simulink model "SimpleCPUCoolingSystem"  (R2024a)
settings: Solver=VariableStepAuto  StartTime=0.0  StopTime=12000  RelTol=1e-3  AbsTol=1e-3  EnableMultiTasking=on
PreLoadFcn:
  | % CPU fan
  | omega_vec = [2000, 2500, 3000]; % Shaft speed vector (rpm)
  | dp_vec = unique([linspace(0, 34.8, 20), 16.1, 24.5]); % Static pressure gain vector (Pa)
  | flow_rate_2000rpm = [
  |    29.0291
  |    26.8708
  |    22.4003
  |    16.0321
  |    11.8087
  |    10.7402
  |    10.3039
  |     9.2101
  |     5.2882
  |     0.001
  |     0.001
  |     0.001
  |     0.001
  |     0.001
  |     0.001
  |     0.001
  |     0.001
  |     0.001
  |     0.001
  |     0.001
  |     0.001
  |     0.001]; % Volumetric flow rate at 2000 rpm (l/min)
  | 
  | flow_rate_2500rpm = [
  |    44.1599
  |    43.4754
  |    41.8968
  |    37.6981
  |    31.3796
  |    25.5726
  |    22.0781
  |    20.5303
  |    19.7231
  |    19.1403
  |    18.9864
  |    17.7518
  |    15.0095
  |     9.9392
  |     3.0478
  |     0.001
  |     0.001
  |     0.001
  |     0.001
  |     0.001
  |     0.001
  |     0.001]; % Volumetric flow rate at 2500 rpm (l/min)
  | 
  | flow_rate_3000rpm = [
  |    62.7057
  |    61.7375
  |    60.1794
  |    58.1656
  |    54.8140
  |    49.9250
  |    43.8984
  |    39.0101
  | ... (+42 lines)
libraries: fl_lib x20, nesl_utility x4, SimscapeFluids_lib x1
(part 2 of 2)

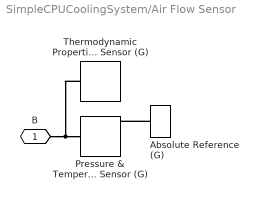
== system SimpleCPUCoolingSystem/Air Flow Sensor ==
  Absolute Reference (G) : fl_lib/Gas/Elements/Absolute Reference (G)
      settings: InternalSimscapePortConfiguration="{\"Bottom\":[],\"Left\":[{\"id\":\"A\",\"label\":\"\",\"type\":\"foundation.gas.gas\"}],\"Right\":[],\"Top\":[]}"
  Pressure & Temperature Sensor (G) : fl_lib/Gas/Sensors/Pressure & Temperature Sensor (G)  reference=foundation.enum.MeasurementReference.difference  pressure=true  pressure_spec=foundation.enum.PressureMeasementSpec.Absolute  temperature=true
      settings: InternalSimscapePortConfiguration="{\"Bottom\":[{\"id\":\"T\",\"label\":\"T\",\"type\":\"output\"}],\"Left\":[{\"id\":\"A\",\"label\":\"A\",\"type\":\"foundation.gas.gas\"}],\"Right\":[{\"id\":\"B\",\"label\":\"B\",\"type\":\"foundation.gas.gas\"},{\"id\":\"P\",\"label\":\"P\",\"type\":\"output\"}],\"Top\":[]}"
  Thermodynamic Properties Sensor (G) : fl_lib/Gas/Sensors/Thermodynamic Properties Sensor (G)  enthalpy=true  density=true  specific_heat=true  entropy=true  s_std=3.8635 kJ/kg/K  p_std=0.101325 MPa  T_std=293.15 K
      settings: InternalSimscapePortConfiguration="{\"Bottom\":[{\"id\":\"CP\",\"label\":\"cp\",\"type\":\"output\"},{\"id\":\"S\",\"label\":\"s\",\"type\":\"output\"}],\"Left\":[{\"id\":\"A\",\"label\":\"A\",\"type\":\"foundation.gas.gas\"}],\"Right\":[{\"id\":\"H\",\"label\":\"h\",\"type\":\"output\"},{\"id\":\"RHO\",\"label\":\"ρ\",\"type\":\"output\"}],\"Top\":[]}"
  B : PMIOPort  Side=Right
  connections:
  Absolute Reference (G)/LConn1 -- Pressure & Temperature Sensor (G)/RConn1
  B/RConn1 -- Thermodynamic Properties Sensor (G)/LConn1 -- Pressure & Temperature Sensor (G)/LConn1

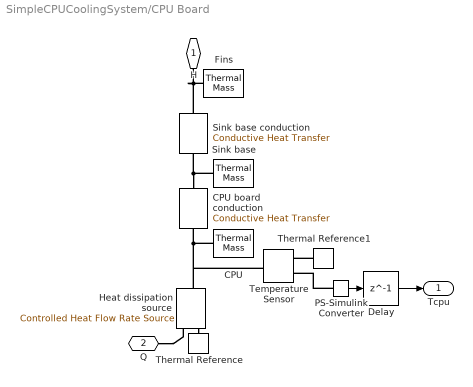
== system SimpleCPUCoolingSystem/CPU Board ==
  CPU : fl_lib/Thermal/Thermal Elements/Thermal Mass  mass_type=foundation.enum.constant_variable.constant  mass=rho_CPU*w_CPU^2*t_CPU g  sp_heat=cp_CPU J/kg/K  mass_min=1e-6 kg  num_ports=foundation.enum.numPorts2.one  m_specify=off  m_priority=High  m=1 kg  m_nominal_specify=off  m_nominal_value=1  m_nominal_unit=kg  T_specify=on  T_priority=High  T=T_init degC  T_nominal_specify=off  T_nominal_value=1  T_nominal_unit=K  Q_specify=off  Q_priority=None  Q=0 W  Q_nominal_specify=off  Q_nominal_value=1  Q_nominal_unit=W
  CPU board conduction : fl_lib/Thermal/Thermal Elements/Conductive Heat Transfer  thermal_type=foundation.enum.ConstantVariableTabulated.Constant  wall_geometry=foundation.enum.ConductionWallGeometry.Planar  area=w_CPU^2 cm^2  thickness=t_CPU cm  d_in=0.05 m  d_out=0.1 m  L=1 m  th_cond_min=10 W/(K*m)  th_cond=k_CPU W/(m*K)  th_cond_TLU=[413, 401, 392, 383, 371, 357, 342] W/(K*m)  temp_TLU=[200, 273, 400, 600, 800, 1000, 1200] K  T_specify=off  T_priority=None  T=0 K  T_nominal_specify=off  T_nominal_value=1  T_nominal_unit=K  Q_specify=off  Q_priority=None  Q=0 W  Q_nominal_specify=off  Q_nominal_value=1  Q_nominal_unit=W
  Delay : Delay  DelayLength=1  InitialCondition=T_init  SampleTime=30
  Fins : fl_lib/Thermal/Thermal Elements/Thermal Mass  mass_type=foundation.enum.constant_variable.constant  mass=rho_HS*N_Fin*t_Fin*h_Fin*l_Fin g  sp_heat=cp_HS J/kg/K  mass_min=1e-6 kg  num_ports=foundation.enum.numPorts2.one  m_specify=off  m_priority=High  m=1 kg  m_nominal_specify=off  m_nominal_value=1  m_nominal_unit=kg  T_specify=on  T_priority=High  T=T_init degC  T_nominal_specify=off  T_nominal_value=1  T_nominal_unit=K  Q_specify=off  Q_priority=None  Q=0 W  Q_nominal_specify=off  Q_nominal_value=1  Q_nominal_unit=W
  Heat dissipation source : fl_lib/Thermal/Thermal Sources/Controlled Heat Flow Rate Source
  PS-Simulink Converter : nesl_utility/PS-Simulink Converter  PhysicalDomain=network_engine_domain  SubClassName=ps_output  LeftPortType=input  RightPortType=output  PseudoPeriodic=off  Frequencies=[]  VectorFormat=1-D array  Unit=degC  AffineConversion=on
  Sink base : fl_lib/Thermal/Thermal Elements/Thermal Mass  mass_type=foundation.enum.constant_variable.constant  mass=rho_HS*w_HS^2*t_HS g  sp_heat=cp_HS J/kg/K  mass_min=1e-6 kg  num_ports=foundation.enum.numPorts2.one  m_specify=off  m_priority=High  m=1 kg  m_nominal_specify=off  m_nominal_value=1  m_nominal_unit=kg  T_specify=on  T_priority=High  T=T_init degC  T_nominal_specify=off  T_nominal_value=1  T_nominal_unit=K  Q_specify=off  Q_priority=None  Q=0 W  Q_nominal_specify=off  Q_nominal_value=1  Q_nominal_unit=W
  Sink base conduction : fl_lib/Thermal/Thermal Elements/Conductive Heat Transfer  thermal_type=foundation.enum.ConstantVariableTabulated.Constant  wall_geometry=foundation.enum.ConductionWallGeometry.Planar  area=N_Fin*l_Fin*t_Fin cm^2  thickness=t_HS cm  d_in=0.05 m  d_out=0.1 m  L=1 m  th_cond_min=10 W/(K*m)  th_cond=k_HS W/(m*K)  th_cond_TLU=[413, 401, 392, 383, 371, 357, 342] W/(K*m)  temp_TLU=[200, 273, 400, 600, 800, 1000, 1200] K  T_specify=off  T_priority=None  T=0 K  T_nominal_specify=off  T_nominal_value=1  T_nominal_unit=K  Q_specify=off  Q_priority=None  Q=0 W  Q_nominal_specify=off  Q_nominal_value=1  Q_nominal_unit=W
  Temperature Sensor : fl_lib/Thermal/Thermal Sensors/Temperature Sensor  temperature_measure=foundation.enum.MeasurementReference.difference
  Thermal Reference : fl_lib/Thermal/Thermal Elements/Thermal Reference
  Thermal Reference1 : fl_lib/Thermal/Thermal Elements/Thermal Reference
  H : PMIOPort  Side=Left
  Q : PMIOPort  Port=2  Side=Right
  Tcpu : Outport  VectorParamsAs1DForOutWhenUnconnected=off
  wires:
  PS-Simulink Converter/1 -> Delay/1
  Delay/1 -> Tcpu/1
  connections:
  CPU/LConn1 -- Temperature Sensor/LConn1 -- Heat dissipation source/LConn1 -- CPU board conduction/LConn1
  Heat dissipation source/RConn2 -- Thermal Reference/LConn1
  Q/RConn1 -- Heat dissipation source/RConn1
  Thermal Reference1/LConn1 -- Temperature Sensor/RConn1
  PS-Simulink Converter/LConn1 -- Temperature Sensor/RConn2
  H/RConn1 -- Sink base conduction/RConn1 -- Fins/LConn1
  Sink base/LConn1 -- CPU board conduction/RConn1 -- Sink base conduction/LConn1

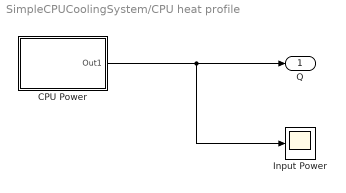
== system SimpleCPUCoolingSystem/CPU heat profile ==
  CPU Power : Subsystem
  Input Power : Scope
  Q : Outport
  wires:
  CPU Power/1(Out1) -> Input Power/1, Q/1

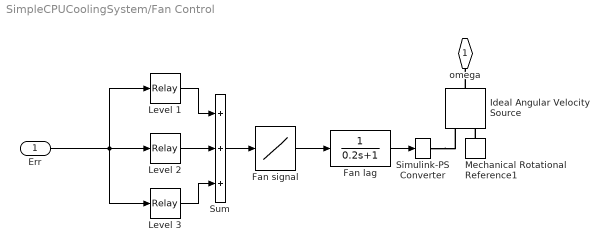
== system SimpleCPUCoolingSystem/Fan Control ==
  Err : Inport
  Fan lag : TransferFcn  Denominator=[0.2 1]
  Fan signal : Lookup_n-D  NumberOfTableDimensions=1  BreakpointsForDimension1=[0, 1, 2 3]  Table=[0, omega_vec(1) omega_vec(2), omega_vec(3)]  InternalRulePriority=Speed  RndMeth=Simplest
  Ideal Angular Velocity Source : fl_lib/Mechanical/Mechanical Sources/Ideal Angular Velocity Source
  Level 1 : Relay  OnSwitchValue=T_level1(2)  OffSwitchValue=T_level1(1)
  Level 2 : Relay  OnSwitchValue=T_level2(2)  OffSwitchValue=T_level2(1)
  Level 3 : Relay  OnSwitchValue=T_level3(2)  OffSwitchValue=T_level3(1)
  Mechanical Rotational Reference1 : fl_lib/Mechanical/Rotational Elements/Mechanical Rotational Reference
  Simulink-PS Converter : nesl_utility/Simulink-PS Converter  PhysicalDomain=network_engine_domain  SubClassName=ps_input  LeftPortType=input  RightPortType=output  PseudoPeriodic=off  Frequencies=[]  NoiseDistribution=none  NoiseParameters=[]  Unit=rpm  AffineConversion=off  FilteringAndDerivatives=zero  SimscapeFilterOrder=1  InputFilterTimeConstant=0.001  UdotUserProvided=1
  Sum : Sum  Inputs=3
  omega : PMIOPort  Side=Right
  wires:
  Fan lag/1 -> Simulink-PS Converter/1
  Level 1/1 -> Sum/1
  Level 2/1 -> Sum/2
  Sum/1 -> Fan signal/1
  Err/1 -> Level 3/1, Level 2/1, Level 1/1
  Fan signal/1 -> Fan lag/1
  Level 3/1 -> Sum/3
  connections:
  Simulink-PS Converter/RConn1 -- Ideal Angular Velocity Source/RConn1
  Mechanical Rotational Reference1/LConn1 -- Ideal Angular Velocity Source/RConn2
  Ideal Angular Velocity Source/LConn1 -- omega/RConn1

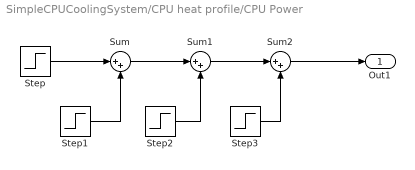
== system SimpleCPUCoolingSystem/CPU heat profile/CPU Power ==
  Step : Step  Time=620  Before=50  After=35  SampleTime=0
  Step1 : Step  Time=4000  After=-25  SampleTime=0
  Step2 : Step  Time=7000  After=35  SampleTime=0
  Step3 : Step  Time=8300  After=-25  SampleTime=0
  Sum : Sum  Inputs=|++
  Sum1 : Sum  Inputs=|++
  Sum2 : Sum  Inputs=|++
  Out1 : Outport
  wires:
  Sum/1 -> Sum1/1
  Step/1 -> Sum/1
  Sum2/1 -> Out1/1
  Step1/1 -> Sum/2
  Step3/1 -> Sum2/2
  Step2/1 -> Sum1/2
  Sum1/1 -> Sum2/1
